simulink model "compensator_tracking_model"  (R2017a)
settings: Solver=VariableStepAuto  StartTime=0.0  StopTime=tf  RelTol=1e-3
undefined symbols (not defined in the file or in its folder): sys, x0, z0
settings Model: Creator=brunolnetto  LastModifiedBy=brunolnetto

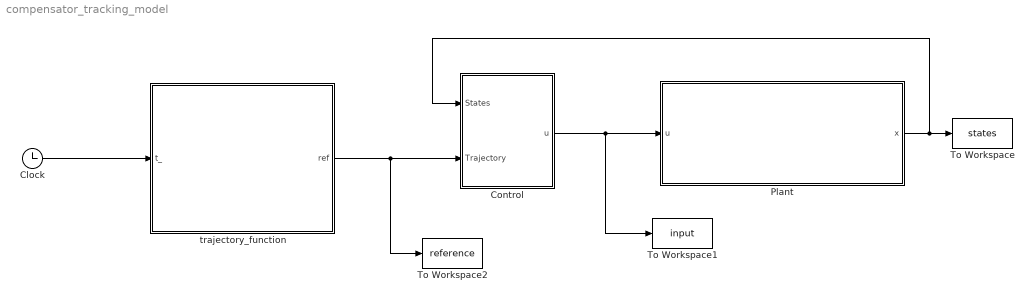
== system compensator_tracking_model ==
  Clock : Clock
  Control : Subsystem
  Plant : Subsystem
      mask Display: image('./plant.png')
  To Workspace : ToWorkspace  VariableName=states  SaveFormat=Structure With Time  SampleTime=-1
  To Workspace1 : ToWorkspace  VariableName=input  SaveFormat=Structure With Time  SampleTime=-1
  To Workspace2 : ToWorkspace  VariableName=reference  SaveFormat=Structure With Time  SampleTime=-1
  trajectory_function : MATLAB Function  TreatAsAtomicUnit=on
  wires:
  Clock/1 -> trajectory_function/1(t_)
  Control/1(u) -> Plant/1(u), To Workspace1/1
  Plant/1(x) -> Control/1(States), To Workspace/1
  trajectory_function/1(ref) -> To Workspace2/1, Control/2(Trajectory)

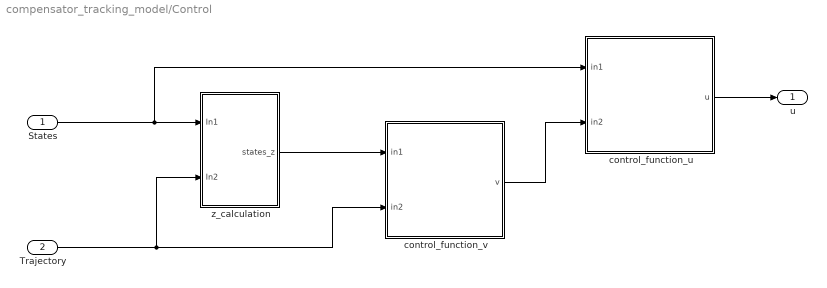
== system compensator_tracking_model/Control ==
  States : Inport
  Trajectory : Inport  Port=2
  control_function_u : MATLAB Function  TreatAsAtomicUnit=on
  control_function_v : MATLAB Function  TreatAsAtomicUnit=on
  z_calculation : Subsystem
  u : Outport
  wires:
  control_function_u/1(u) -> u/1
  Trajectory/1 -> z_calculation/2(In2), control_function_v/2(in2)
  States/1 -> control_function_u/1(in1), z_calculation/1(In1)
  z_calculation/1(states_z) -> control_function_v/1(in1)
  control_function_v/1(v) -> control_function_u/2(in2)

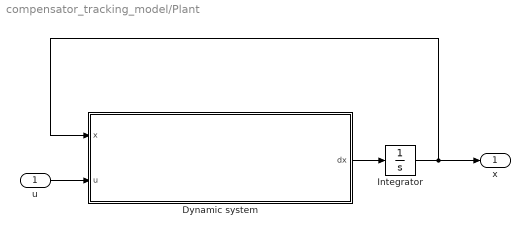
== system compensator_tracking_model/Plant ==
  u : Inport
  Dynamic system : Subsystem
      mask Display: image('./plant.png')
  Integrator : Integrator  InitialCondition=x0
  x : Outport
  wires:
  Dynamic system/1(dx) -> Integrator/1
  u/1 -> Dynamic system/2(u)
  Integrator/1 -> x/1, Dynamic system/1(x)

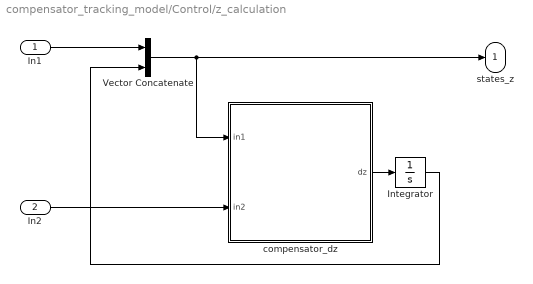
== system compensator_tracking_model/Control/z_calculation ==
  In1 : Inport
  In2 : Inport  Port=2
  Integrator : Integrator  InitialCondition=z0
  Vector Concatenate : Concatenate
  compensator_dz : MATLAB Function  TreatAsAtomicUnit=on
  states_z : Outport
  wires:
  In1/1 -> Vector Concatenate/1
  In2/1 -> compensator_dz/2(in2)
  Integrator/1 -> Vector Concatenate/2
  compensator_dz/1(dz) -> Integrator/1
  Vector Concatenate/1 -> states_z/1, compensator_dz/1(in1)

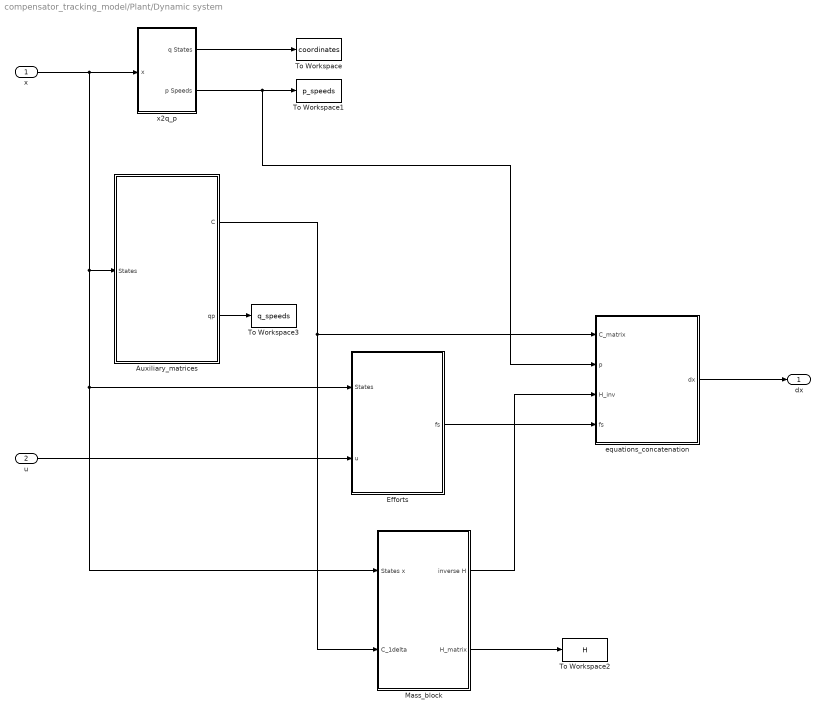
== system compensator_tracking_model/Plant/Dynamic system ==
  x : Inport
  u : Inport  Port=2
  Auxiliary_matrices : Subsystem
  Efforts : Subsystem
  Mass_block : Subsystem
  To Workspace : ToWorkspace  VariableName=coordinates  SaveFormat=Structure With Time  SampleTime=-1
  To Workspace1 : ToWorkspace  VariableName=p_speeds  SaveFormat=Structure With Time  SampleTime=-1
  To Workspace2 : ToWorkspace  VariableName=H  SaveFormat=Structure With Time  SampleTime=-1
  To Workspace3 : ToWorkspace  VariableName=q_speeds  SaveFormat=Structure With Time  SampleTime=-1
  equations_concatenation : Subsystem
  x2q_p : Subsystem
  dx : Outport
  wires:
  Auxiliary_matrices/1(C) -> Mass_block/2("C_1delta  "), equations_concatenation/1(C_matrix)
  Auxiliary_matrices/2(qp) -> To Workspace3/1
  x2q_p/2(p Speeds) -> To Workspace1/1, equations_concatenation/2(p)
  x2q_p/1(q States) -> To Workspace/1
  Efforts/1(fs) -> equations_concatenation/4(fs)
  Mass_block/1(inverse H) -> equations_concatenation/3(H_inv)
  equations_concatenation/1(dx) -> dx/1
  u/1 -> Efforts/2(u)
  x/1 -> x2q_p/1(x), Efforts/1(States), Mass_block/1(States x), Auxiliary_matrices/1(States)
  Mass_block/2(H_matrix) -> To Workspace2/1

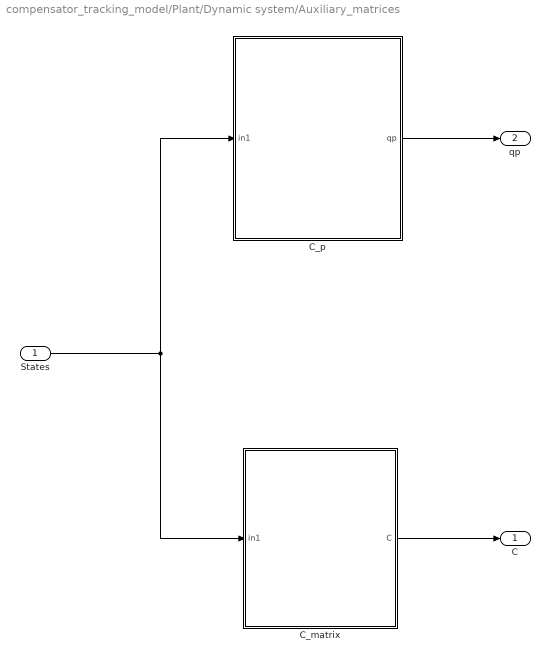
== system compensator_tracking_model/Plant/Dynamic system/Auxiliary_matrices ==
  States : Inport
  C_matrix : MATLAB Function  TreatAsAtomicUnit=on
  C_p : MATLAB Function  TreatAsAtomicUnit=on
  C : Outport
  qp : Outport  Port=2
  wires:
  C_matrix/1(C) -> C/1
  States/1 -> C_p/1(in1), C_matrix/1(in1)
  C_p/1(qp) -> qp/1

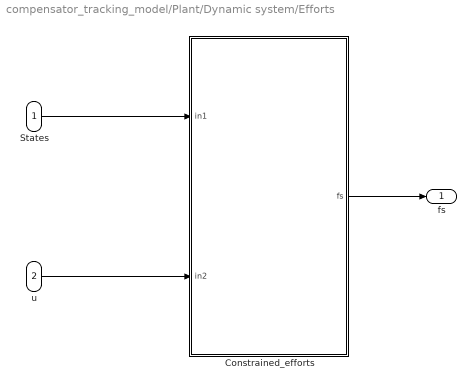
== system compensator_tracking_model/Plant/Dynamic system/Efforts ==
  States : Inport
  u : Inport  Port=2
  Constrained_efforts : MATLAB Function  TreatAsAtomicUnit=on
  fs : Outport
  wires:
  States/1 -> Constrained_efforts/1(in1)
  u/1 -> Constrained_efforts/2(in2)
  Constrained_efforts/1(fs) -> fs/1

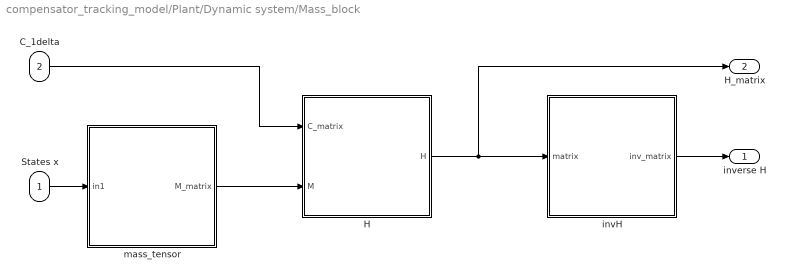
== system compensator_tracking_model/Plant/Dynamic system/Mass_block ==
  States x : Inport
  "C_1delta  " : Inport  Port=2
  H : MATLAB Function  TreatAsAtomicUnit=on
  invH : MATLAB Function  TreatAsAtomicUnit=on
  mass_tensor : MATLAB Function  TreatAsAtomicUnit=on
  inverse H : Outport
  H_matrix : Outport  Port=2
  wires:
  States x/1 -> mass_tensor/1(in1)
  "C_1delta  "/1 -> H/1(C_matrix)
  invH/1(inv_matrix) -> inverse H/1
  H/1(H) -> invH/1(matrix), H_matrix/1
  mass_tensor/1(M_matrix) -> H/2(M)

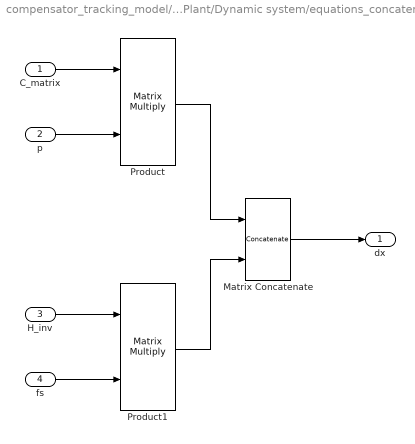
== system compensator_tracking_model/Plant/Dynamic system/equations_concatenation ==
  C_matrix : Inport
  p : Inport  Port=2
  H_inv : Inport  Port=3
  fs : Inport  Port=4
  Matrix Concatenate : Concatenate  ConcatenateDimension=2
  Product : Product  Multiplication=Matrix(*)
  Product1 : Product  Multiplication=Matrix(*)
  dx : Outport
  wires:
  Product/1 -> Matrix Concatenate/1
  p/1 -> Product/2
  C_matrix/1 -> Product/1
  Product1/1 -> Matrix Concatenate/2
  H_inv/1 -> Product1/1
  fs/1 -> Product1/2
  Matrix Concatenate/1 -> dx/1

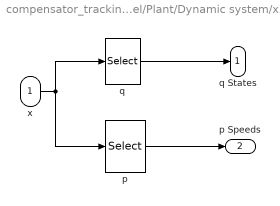
== system compensator_tracking_model/Plant/Dynamic system/x2q_p ==
  x : Inport
  p : Selector  InputPortWidth=length(sys.kin.q) + length(sys.kin.p{end})  IndexOptions=Index vector (dialog)  Indices=(length(sys.kin.q))+1:(length(sys.kin.q) + length(sys.kin.p{end}))  OutputSizes=1
  q : Selector  InputPortWidth=length(sys.kin.q) + length(sys.kin.p{end})  IndexOptions=Index vector (dialog)  Indices=1:length(sys.kin.q)  OutputSizes=1
  q States : Outport
  p Speeds : Outport  Port=2
  wires:
  x/1 -> p/1, q/1
  q/1 -> q States/1
  p/1 -> p Speeds/1

== matlab function compensator_tracking_model/Control/control_function_v ==
  data: in1 input; v output size=size(v_); in2 input
function v = control_function_v(in1,in2)

%    This function was generated by the Symbolic Math Toolbox version 7.2.

%    20-Feb-2021 19:35:54



x_1 = in1(1,:);

x_2 = in1(2,:);

x_3 = in1(3,:);

x_4 = in1(4,:);

x_5 = in1(5,:);

x_6 = in1(6,:);

x_pos_ref = in2(1,:);

xp_ref = in2(3,:);

xpp_ref = in2(5,:);

xppp_ref = in2(7,:);

y_pos_ref = in2(2,:);

yp_ref = in2(4,:);

ypp_ref = in2(6,:);

yppp_ref = in2(8,:);

t2 = cos(x_3);

t3 = sin(x_3);

v = [x_6;(t2.*x_2.*-1.220807155376085e1+t3.*x_1.*1.220807155376085e1-t3.*x_pos_ref.*1.220807155376085e1-t3.*xp_ref.*1.590569433143519e1-t3.*xpp_ref.*6.907755278982137-t3.*xppp_ref.*1.0+t2.*y_pos_ref.*1.220807155376085e1+t2.*yp_ref.*1.590569433143519e1+t2.*ypp_ref.*6.907755278982137+t2.*yppp_ref.*1.0-x_4.*x_5.*6.907755278982137-x_5.*x_6.*2.0)./x_4];

end

== matlab function compensator_tracking_model/Plant/Dynamic system/Mass_block/mass_tensor ==
  data: in1 input; M_matrix output
function M_matrix = Mass_matrix(in1)

%    This function was generated by the Symbolic Math Toolbox version 7.2.

%    12-Dec-2021 17:12:14



phi1 = in1(4,:);

phi2 = in1(5,:);

phi3 = in1(6,:);

th = in1(3,:);

t2 = cos(phi1);

t3 = cos(phi2);

t4 = cos(phi3);

t5 = cos(th);

t6 = sin(th);

M_matrix = reshape([4.22e-1,0.0,0.0,0.0,0.0,0.0,0.0,4.22e-1,0.0,0.0,0.0,0.0,0.0,0.0,t2.^2.*2.518133623269337e-7+t3.^2.*2.518133623269337e-7+t4.^2.*2.518133623269337e-7+t5.^2.*1.3875e-2+t6.^2.*1.3875e-2+2.520833333333333e-4,0.0,0.0,0.0,0.0,0.0,0.0,0.0,0.0,0.0,0.0,0.0,0.0,0.0,0.0,0.0,0.0,0.0,0.0,0.0,0.0,0.0],[6,6]);

end

== matlab function compensator_tracking_model/Plant/Dynamic system/Auxiliary_matrices/C_matrix ==
  data: in1 input; C output
function C = ConstraintMatrix(in1)

%    This function was generated by the Symbolic Math Toolbox version 7.2.

%    12-Dec-2021 17:12:14



th = in1(3,:);

t2 = cos(th);

t3 = sin(th);

t4 = t3.*-5.813953488372093;

t5 = t2.*5.813953488372093;

C = reshape([1.0,0.0,0.0,t3.*1.162790697674419e1,t2.*1.007006283470277e1+t4,t2.*-1.007006283470277e1+t4,0.0,1.0,0.0,t2.*-1.162790697674419e1,t3.*1.007006283470277e1+t5,t3.*-1.007006283470277e1+t5,0.0,0.0,1.0,-2.906976744186047,-2.906976744186047,-2.906976744186047],[6,3]);

end

== matlab function compensator_tracking_model/trajectory_function ==
  data: t_ input; ref output
function ref = trajectory_generator(t_)

%    This function was generated by the Symbolic Math Toolbox version 7.2.

%    10-Feb-2021 17:47:43



t2 = t_.*3.0;

t3 = cos(t2);

t4 = sin(t_);

t5 = t3.*t4;

t6 = cos(t_);

t7 = t3.*t6;

t8 = sin(t2);

ref = [t7;t5;-t5-t6.*t8.*3.0;t7-t4.*t8.*3.0;t3.*t6.*-1.0e1+t4.*t8.*6.0;t3.*t4.*-1.0e1-t6.*t8.*6.0;t3.*t4.*2.8e1+t6.*t8.*3.6e1;t3.*t6.*-2.8e1+t4.*t8.*3.6e1];

end

== matlab function compensator_tracking_model/Control/control_function_u ==
  data: in1 input; u output size=size(u); in2 input
function u = control_function_u(in1,in2)

%    This function was generated by the Symbolic Math Toolbox version 7.2.

%    20-Feb-2021 19:35:55



v1 = in2(1,:);

v2 = in2(2,:);

x_3 = in1(3,:);

t2 = cos(x_3);

t3 = sin(x_3);

t4 = t2.^2;

t5 = t3.^2;

t6 = t4+t5;

t7 = t6.*v1.*1.65e-2;

u = [t7+v2.*2.151974637681159e-3;t7-v2.*2.151974637681159e-3];

end

== matlab function compensator_tracking_model/Plant/Dynamic system/Efforts/Constrained_efforts ==
  data: in1 input; fs output; in2 input
function fs = ConstrainedEffort(in1,in2)

%    This function was generated by the Symbolic Math Toolbox version 7.2.

%    12-Dec-2021 17:12:14



p1 = in1(7,:);

p2 = in1(8,:);

p3 = in1(9,:);

phi1 = in1(4,:);

phi2 = in1(5,:);

phi3 = in1(6,:);

tau1 = in2(1,:);

tau2 = in2(2,:);

tau3 = in2(3,:);

th = in1(3,:);

t2 = cos(th);

t3 = sin(th);

t4 = p3.^2;

t5 = cos(phi2);

t6 = sin(phi2);

t7 = cos(phi3);

t8 = sin(phi3);

t9 = cos(phi1);

t10 = sin(phi1);

fs = [t2.*tau2.*1.007006283470277e1+t3.*tau1.*1.162790697674419e1-t2.*tau3.*1.007006283470277e1-t3.*tau2.*5.813953488372093-t3.*tau3.*5.813953488372093-t2.*t4.*t5.*t6.*2.535776381249999e-6+t3.*t4.*t5.*t6.*1.464031176319382e-6+t2.*t4.*t7.*t8.*2.535776381249999e-6+t3.*t4.*t7.*t8.*1.464031176319382e-6-t3.*t4.*t9.*t10.*2.928062352638764e-6;t2.*tau1.*-1.162790697674419e1+t2.*tau2.*5.813953488372093+t2.*tau3.*5.813953488372093+t3.*tau2.*1.007006283470277e1-t3.*tau3.*1.007006283470277e1-t2.*t4.*t5.*t6.*1.464031176319382e-6-t3.*t4.*t5.*t6.*2.535776381249999e-6-t2.*t4.*t7.*t8.*1.464031176319382e-6+t3.*t4.*t7.*t8.*2.535776381249999e-6+t2.*t4.*t9.*t10.*2.928062352638764e-6;tau1.*-2.906976744186047-tau2.*2.906976744186047-tau3.*2.906976744186047-t2.*t3.*t4.*1.434929627468613e-42-t4.*t5.*t6.*7.32015588159691e-7-t4.*t7.*t8.*7.32015588159691e-7-t4.*t9.*t10.*7.32015588159691e-7+p1.*p3.*t2.*t5.*t6.*5.071552762499998e-6-p1.*p3.*t3.*t5.*t6.*2.928062352638764e-6+p2.*p3.*t2.*t5.*t6.*2.928062352638764e-6+p2.*p3.*t3.*t5.*t6.*5.071552762499998e-6-p1.*p3.*t2.*t7.*t8.*5.071552762499998e-6-p1.*p3.*t3.*t7.*t8.*2.928062352638764e-6+p2.*p3.*t2.*t7.*t8.*2.928062352638764e-6-p2.*p3.*t3.*t7.*t8.*5.071552762499998e-6+p1.*p3.*t3.*t9.*t10.*5.856124705277528e-6-p2.*p3.*t2.*t9.*t10.*5.856124705277528e-6];

end

== matlab function compensator_tracking_model/Control/z_calculation/compensator_dz ==
  data: in1 input; dz output; in2 input
function dz = compensator_dz(in1,in2)

%    This function was generated by the Symbolic Math Toolbox version 7.2.

%    20-Feb-2021 19:35:54



x_1 = in1(1,:);

x_2 = in1(2,:);

x_3 = in1(3,:);

x_4 = in1(4,:);

x_5 = in1(5,:);

x_6 = in1(6,:);

x_pos_ref = in2(1,:);

xp_ref = in2(3,:);

xpp_ref = in2(5,:);

xppp_ref = in2(7,:);

y_pos_ref = in2(2,:);

yp_ref = in2(4,:);

ypp_ref = in2(6,:);

yppp_ref = in2(8,:);

t2 = cos(x_3);

t3 = sin(x_3);

dz = x_4.*-1.590569433143519e1-x_6.*6.907755278982137-t2.*x_1.*1.220807155376085e1-t3.*x_2.*1.220807155376085e1+t2.*x_pos_ref.*1.220807155376085e1+t2.*xp_ref.*1.590569433143519e1+t2.*xpp_ref.*6.907755278982137+t2.*xppp_ref+t3.*y_pos_ref.*1.220807155376085e1+t3.*yp_ref.*1.590569433143519e1+t3.*ypp_ref.*6.907755278982137+t3.*yppp_ref+x_4.*x_5.^2;

end

== matlab function compensator_tracking_model/Plant/Dynamic system/Mass_block/H ==
  data: C_matrix input; H output; M input
function H = ConstrinedMassMatrix(C_matrix, M)
% MASSMATRIX
%    This function was generated by the Symbolic Math Toolbox version 7.2.
%    16-Oct-2020 11:55:07

    H = C_matrix'*M*C_matrix;
end

== matlab function compensator_tracking_model/Plant/Dynamic system/Mass_block/invH ==
  data: matrix input; inv_matrix output
function inv_matrix = matrix_inverse(matrix)
% MASSMATRIX
%    This function was generated by the Symbolic Math Toolbox version 7.2.
%    16-Oct-2020 11:55:07

    inv_matrix = inv(matrix);
end

== matlab function compensator_tracking_model/Plant/Dynamic system/Auxiliary_matrices/C_p ==
  data: in1 input; qp output
function qp = KinematicVector(in1)

%    This function was generated by the Symbolic Math Toolbox version 7.2.

%    12-Dec-2021 17:12:14



p1 = in1(7,:);

p2 = in1(8,:);

p3 = in1(9,:);

th = in1(3,:);

t2 = p3.*-2.906976744186047;

t3 = cos(th);

t4 = sin(th);

t5 = p2.*t3.*5.813953488372093;

t6 = p1.*t4.*-5.813953488372093;

qp = [p1;p2;p3;t2+p1.*t4.*1.162790697674419e1-p2.*t3.*1.162790697674419e1;t2+t5+t6+p1.*t3.*1.007006283470277e1+p2.*t4.*1.007006283470277e1;t2+t5+t6-p1.*t3.*1.007006283470277e1-p2.*t4.*1.007006283470277e1];

end
